simulink model "ctrl_TT"  (R2022b)
settings: Solver=FixedStepAuto  StartTime=0.0  StopTime=Tf  FixedStep=0.05  RelTol=1e-3
InitFcn:
  | run;
StopFcn:
  | save('testdata')
undefined symbols (not defined in the file): Ba_0, Bb, Bv_0, Bx_0, Cp, Cp_prime, d, dA_BP1, dA_BP2, dA_Hull, dA_PH, dA_Sail, dA_SProot, dA_X1a, dA_X1b, dA_X2a, dA_X2b, dA_X3a, dA_X3b, dA_X4a, dA_X4b, Ixx, Ixy, Ixz, Iyy, Iyz, Izz, Mb, n_BP1, n_BP2, n_Hull, n_PH, n_Sail, n_SProot, n_X2a, n_X2b, n_X3a, n_X4a, n_X4b, nt_BP1, nt_BP2, nt_Hull, nt_PH, nt_Sail, nt_SProot, nt_X1a, nt_X1b, nt_X2a, nt_X2b, nt_X3a, nt_X3b, nt_X4a, nt_X4b, Seastate, Tf, vt1_BP1, vt1_BP2, vt1_Hull, vt1_PH, vt1_Sail ... (+44)
libraries: simulink x8, sharedtransform x2, dspmathops x2
(part 1 of 5)
settings Model: Creator=yagkim  LastModifiedBy=maclin
settings SolverCC: AlgebraicLoopSolver=TrustRegion
settings DebuggingCC: UnconnectedInputMsg=warning  UnconnectedOutputMsg=warning  UnconnectedLineMsg=warning  SFMachineParentedDataDiag=warning  ArithmeticOperatorsInVariantConditions=warning
settings ModelReferenceCC: EnableRefExpFcnMdlSchedulingChecks=on
settings SFSimCC: CustomCodeUndefinedFunction=UseInterfaceOnly
settings RTWCC: DLArmComputeVersion=19.05

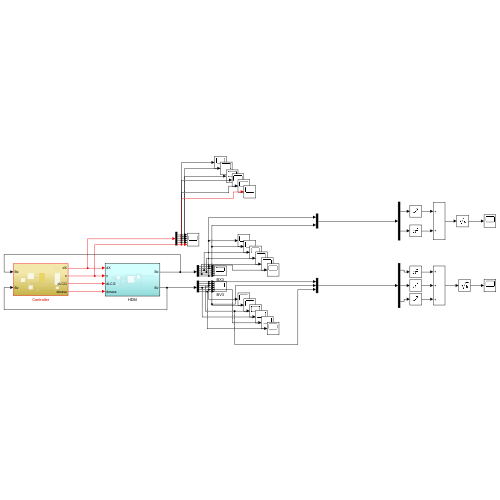
[thumbnail: Simulink's stored preview of the top-level diagram]
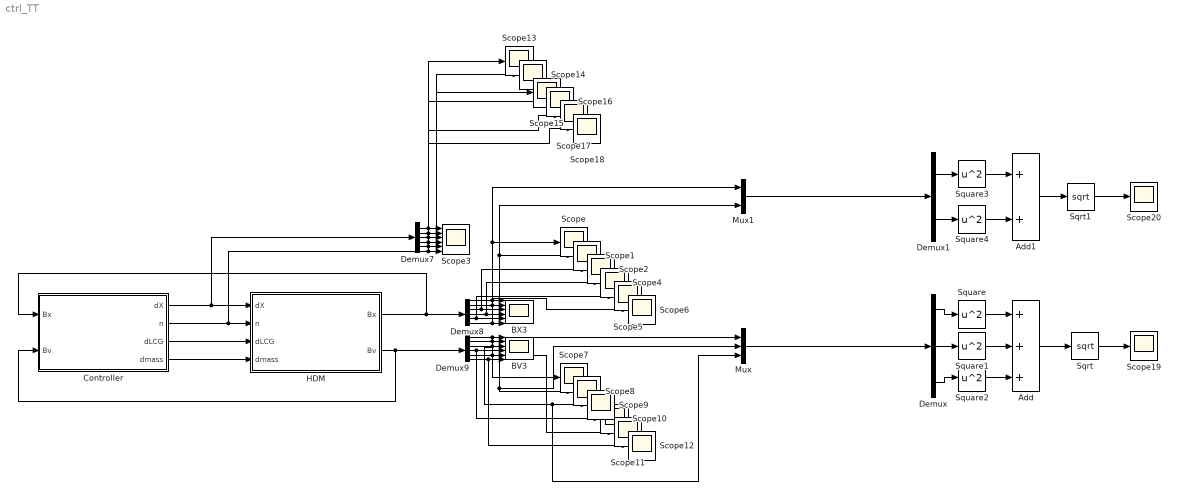
== system ctrl_TT ==
  Add : Sum  Inputs=+++
  Add1 : Sum
  BV3 : Scope  NumInputPorts=6
  BX3 : Scope  NumInputPorts=6
  Controller : Subsystem
  Demux : Demux  Outputs=3
  Demux1 : Demux  Outputs=2
  Demux7 : Demux  Outputs=5
  Demux8 : Demux  Outputs=6
  Demux9 : Demux  Outputs=6
  HDM : Subsystem
  Mux : Mux  Inputs=3
  Mux1 : Mux  Inputs=2
  Scope{,1..2,4..20} (20 alike) : Scope
  Scope3 : Scope  NumInputPorts=6
  Sqrt : Sqrt
  Sqrt1 : Sqrt
  Square{,1..4} (5 alike) : Math  Operator=square
  wires:
  Demux7/1 -> Scope13/1, Scope3/1
  Demux7/5 -> Scope17/1, Scope3/5
  Demux7/4 -> Scope16/1, Scope3/4
  Demux7/3 -> Scope15/1, Scope3/3
  Demux7/2 -> Scope14/1, Scope3/2
  Controller/4(dmass) -> HDM/4(dmass)
  Controller/3(dLCG) -> HDM/3(dLCG)
  Controller/1(dX) -> HDM/1(dX), Demux7/1
  Controller/2(n) -> HDM/2(n), Scope18/1, Scope3/6
  Demux8/1 -> Scope/1, Mux1/1, BX3/1
  Demux8/2 -> Scope1/1, Mux1/2, BX3/2
  Demux9/3 -> Mux/3, Scope9/1, BV3/3
  Demux8/3 -> BX3/3, Scope2/1
  Demux9/1 -> Mux/1, BV3/1, Scope7/1
  Demux8/4 -> BX3/4, Scope4/1
  Demux9/5 -> Scope11/1, BV3/5
  Demux8/6 -> Scope6/1, BX3/6
  Demux9/2 -> Mux/2, Scope8/1, BV3/2
  Demux8/5 -> BX3/5, Scope5/1
  Demux9/6 -> Scope12/1, BV3/6
  HDM/2(Bv) -> Controller/2(Bv), Demux9/1
  Demux9/4 -> BV3/4, Scope10/1
  HDM/1(Bx) -> Demux8/1, Controller/1(Bx)
  Add/1 -> Sqrt/1
  Square/1 -> Add/1
  Demux/1 -> Square/1
  Demux/3 -> Square2/1
  Sqrt/1 -> Scope19/1
  Square1/1 -> Add/2
  Square2/1 -> Add/3
  Demux/2 -> Square1/1
  Mux/1 -> Demux/1
  Square4/1 -> Add1/2
  Mux1/1 -> Demux1/1
  Sqrt1/1 -> Scope20/1
  Demux1/2 -> Square4/1
  Add1/1 -> Sqrt1/1
  Demux1/1 -> Square3/1
  Square3/1 -> Add1/1

== system ctrl_TT/Controller ==
  Bx : Inport
  Bv : Inport  Port=2
  Clock : Clock
  Constant : Constant  Value=[-1 0 0 0 0 0; 0 -1 0 0 0 0; 0 0 1 0 0 0; 0 0 0 1 0 0; 0 0 0 0 1 0; 0 0 0 0 0 1]
  Constant1 : Constant  Value=0
  Constant2 : Constant  Value=[-1 0 0 0 0 0; 0 -1 0 0 0 0; 0 0 1 0 0 0; 0 0 0 1 0 0; 0 0 0 0 1 0; 0 0 0 0 0 1]
  FF velocity ctrl : MATLAB Function  TreatAsAtomicUnit=on
  MATLAB Function2 : MATLAB Function  TreatAsAtomicUnit=on
  Marin PID : MATLAB Function  TreatAsAtomicUnit=on
  Matrix Multiply : Product  Multiplication=Matrix(*)
  Matrix Multiply1 : Product  Multiplication=Matrix(*)
  Scope : Scope
  Scope1 : Scope
  Selector1 : Selector  InputPortWidth=6  IndexOptions=Index vector (dialog)  Indices=[1 2 3]  OutputSizes=1
  Subsystem1 : Subsystem
  dX : Outport
  n : Outport  Port=2
  dLCG : Outport  Port=3
  dmass : Outport  Port=4
  wires:
  Subsystem1/1(z_d) -> Marin PID/1(z_ref)
  FF velocity ctrl/1(n) -> n/1
  Subsystem1/3(v) -> FF velocity ctrl/1(v_ref), Scope/1
  Marin PID/1(dX) -> dX/1
  Constant1/1 -> dLCG/1, dmass/1
  MATLAB Function2/1(pd) -> Scope1/1, Subsystem1/1(pd(t))
  MATLAB Function2/2(pdp) -> Subsystem1/2(pd(t)')
  Subsystem1/2(psi_d) -> Marin PID/2(psi_ref)
  Bx/1 -> Matrix Multiply/2
  Selector1/1 -> Subsystem1/3(p)
  Clock/1 -> MATLAB Function2/1(time)
  Matrix Multiply/1 -> Selector1/1, Marin PID/4(Bx)
  Constant/1 -> Matrix Multiply/1
  Bv/1 -> Matrix Multiply1/2
  Matrix Multiply1/1 -> Marin PID/3(Bv)
  Constant2/1 -> Matrix Multiply1/1

== system ctrl_TT/HDM ==
  dX : Inport
  n : Inport  Port=2
  dLCG : Inport  Port=3
  dmass : Inport  Port=4
  Constant1 : Constant  Value=Seastate
  HDM B3 : Subsystem  InitFcn='main'
  Integration and Coord. Transfrom : Subsystem
  Scope : Scope
  Scope1 : Scope
  actuator saturation : Subsystem
  Bx : Outport
  Bv : Outport  Port=2
  wires:
  actuator saturation/4(dmass (kg)) -> HDM B3/4(dmass), Scope1/1
  actuator saturation/3(dLCG (m)) -> HDM B3/3(dLCG)
  actuator saturation/2(n) -> HDM B3/2(n)
  actuator saturation/1(dX) -> HDM B3/1(dX CTRL)
  dmass/1 -> actuator saturation/4(dmass), Scope/1
  dLCG/1 -> actuator saturation/3(dLCG)
  n/1 -> actuator saturation/2("n ")
  dX/1 -> actuator saturation/1("dX ")
  Constant1/1 -> HDM B3/8(SeaState)
  HDM B3/1(F_hyd) -> Integration and Coord. Transfrom/2(F_hyd)
  Integration and Coord. Transfrom/3(Ba) -> HDM B3/7(Ba)
  Integration and Coord. Transfrom/1("Bx ") -> Bx/1, HDM B3/5(Bx), Integration and Coord. Transfrom/1(Bx)
  Integration and Coord. Transfrom/2(Bv) -> Bv/1, HDM B3/6(Bv)

== system ctrl_TT/Controller/Subsystem1 ==
  pd(t) : Inport
  pd(t)' : Inport  Port=2
  p : Inport  Port=3
  1,1 : Selector  NumberOfDimensions=2  InputPortWidth=3  IndexOptions=Index vector (dialog),Index vector (dialog)  Indices=1,1  OutputSizes=1,1
  2,1 : Selector  NumberOfDimensions=2  InputPortWidth=3  IndexOptions=Index vector (dialog),Index vector (dialog)  Indices=2,1  OutputSizes=1,1
  Add1 : Sum
  Demux3 : Demux  Outputs=3
  Derivative : Derivative
  Direction Cosine Matrix to Rotation Angles : sharedtransform/Direction Cosine Matrix to Rotation Angles  rotationOrder=ZYX  aMode=aMode  action=None  tolerance=eps(2)
      settings: LibrarySourceBlock=|
      | aerolibtransform2/Direction Cosine Matrix
      | to Rotation Angles
  Display{,1..7} (8 alike) : Display
  Dot Product1 : DotProduct  OutDataTypeStr=Inherit: Inherit via internal rule
  Gain : Gain  Gain=-1
  Gain1 : Gain  Gain=0.1
  MATLAB Function : MATLAB Function  TreatAsAtomicUnit=on
  Matrix Multiply1 : Product  Multiplication=Matrix(*)
  Mux1 : Mux  Inputs=2
  Scope : Scope
  Scope1 : Scope
  Selector : Selector  InputPortWidth=3  IndexOptions=Index vector (dialog)  Indices=[1 2]  OutputSizes=1
  Selector1 : Selector  InputPortWidth=3  IndexOptions=Index vector (dialog)  Indices=[1 2]  OutputSizes=1
  Subsystem1 : Subsystem
  Subsystem2 : Subsystem
  Subsystem3 : Subsystem
  Sum : Sum  Inputs=|+-
  Terminator3 : Terminator
  Terminator4 : Terminator
  z_d : Outport
  psi_d : Outport  Port=2
  v : Outport  Port=3
  wires:
  pd(t)'/1 -> Subsystem2/2(pd(y)'), Subsystem1/1(pd(t)'), Selector1/1
  pd(t)/1 -> Derivative/1, Sum/1, Subsystem2/1(pd(y))
  p/1 -> Sum/2, Subsystem2/3(p)
  Subsystem2/1(RTI) -> Matrix Multiply1/1, Display4/1
  2,1/1 -> Mux1/2
  1,1/1 -> Mux1/1
  Subsystem2/3(zd) -> z_d/1
  Gain/1 -> Display/1, psi_d/1
  Subsystem2/2(RWT) -> Matrix Multiply1/2
  Sum/1 -> Display6/1, Scope/1, Selector/1
  Derivative/1 -> Subsystem3/1(In1)
  Subsystem3/1(Out1) -> Scope1/1
  Gain1/1 -> Add1/1
  Add1/1 -> Dot Product1/1
  Mux1/1 -> Dot Product1/2
  Dot Product1/1 -> Display3/1, v/1
  Selector/1 -> Display5/1, Gain1/1
  Selector1/1 -> Add1/2
  Subsystem1/1(Out1) -> Display2/1
  Direction Cosine Matrix to Rotation Angles/1 -> Demux3/1
  Matrix Multiply1/1 -> MATLAB Function/1(u), Display7/1, 2,1/1, 1,1/1
  MATLAB Function/1(y) -> Display1/1, Direction Cosine Matrix to Rotation Angles/1
  Demux3/2 -> Terminator3/1
  Demux3/3 -> Terminator4/1
  Demux3/1 -> Gain/1

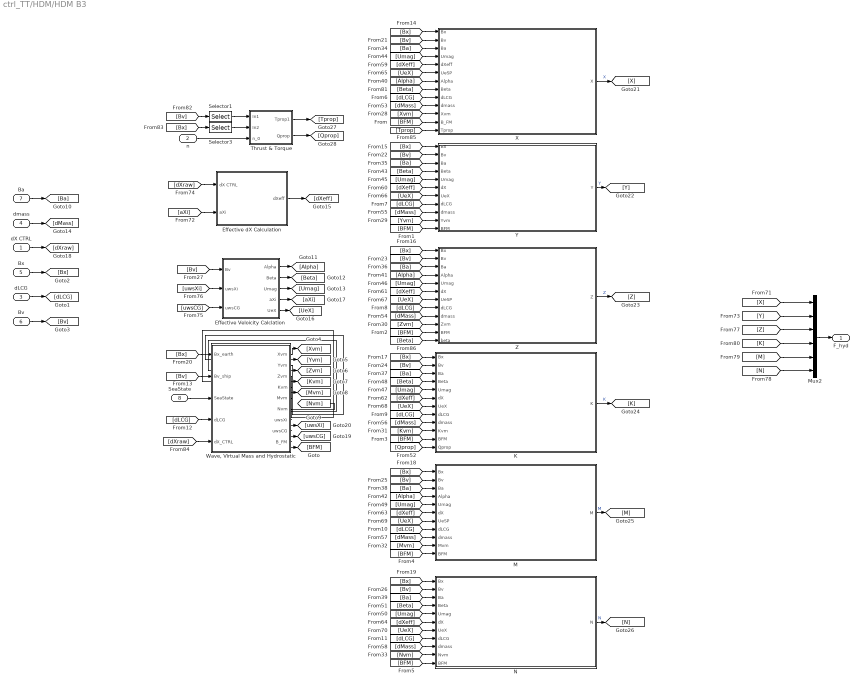
== system ctrl_TT/HDM/HDM B3 ==
  dX CTRL : Inport
  n : Inport  Port=2
  dLCG : Inport  Port=3
  dmass : Inport  Port=4
  Bx : Inport  Port=5
  Bv : Inport  Port=6
  Ba : Inport  Port=7
  SeaState : Inport  Port=8
  Effective Veloicity Calclation : Subsystem
  Effective dX Calculation : Subsystem
  K : Subsystem
  M : Subsystem
  Mux2 : Mux  Inputs=6
  N : Subsystem
  Selector1 : Selector  InputPortWidth=6  IndexOptions=Index vector (dialog)  Indices=1  OutputSizes=1
  Selector3 : Selector  InputPortWidth=6  IndexOptions=Index vector (dialog)  Indices=3  OutputSizes=1
  Thrust & Torque : Subsystem
  "Wave, Virtual Mass and Hydrostatic" : Subsystem
  X : Subsystem
  Y : Subsystem
  Z : Subsystem
  F_hyd : Outport  VectorParamsAs1DForOutWhenUnconnected=off
  wires:
  Z/1(Z) -> [Z]  "Z"
  [Beta] -> Z/12(beta)
  Thrust & Torque/2(Qprop) -> [Qprop]
  [Tprop] -> X/13(Tprop)
  Thrust & Torque/1(Tprop1) -> [Tprop]
  [Bx] -> Selector3/1
  Selector3/1 -> Thrust & Torque/2(In2)
  Selector1/1 -> Thrust & Torque/1(In1)
  [Bv] -> Selector1/1
  [Qprop] -> K/12(Qprop)
  [N] -> Mux2/6
  [M] -> Mux2/5
  [K] -> Mux2/4
  [Z] -> Mux2/3
  [Y] -> Mux2/2
  [X] -> Mux2/1
  [dXraw] -> "Wave, Virtual Mass and Hydrostatic"/5(dX_CTRL)
  [Beta] -> X/8(Beta)
  N/1(N) -> [N]  "N"
  M/1(M) -> [M]  "M"
  K/1(K) -> [K]  "K"
  Y/1(Y) -> [Y]  "Y"
  X/1(X) -> [X]  "X"
  [uwsXi] -> Effective Veloicity Calclation/2(uwsXi)
  "Wave, Virtual Mass and Hydrostatic"/7(uwsXi) -> [uwsXi]
  [uwsCG] -> Effective Veloicity Calclation/3(uwsCG)
  "Wave, Virtual Mass and Hydrostatic"/8(uwsCG) -> [uwsCG]
  [dXraw] -> Effective dX Calculation/1(dX CTRL)
  dX CTRL/1 -> [dXraw]
  [aXi] -> Effective dX Calculation/2(aXi)
  Effective Veloicity Calclation/4(aXi) -> [aXi]
  [UeX] -> N/7(UeX)
  [UeX] -> M/7(UeSP)
  [UeX] -> K/7(UeX)
  [UeX] -> Z/7(UeSP)
  [UeX] -> Y/7(UeX)
  [UeX] -> X/6(UeSP)
  Effective Veloicity Calclation/5(UeX) -> [UeX]
  [dXeff] -> N/6(dX)
  [dXeff] -> M/6(dX)
  [dXeff] -> K/6(dX)
  [dXeff] -> Z/6(dX)
  [dXeff] -> Y/6(dX)
  [dXeff] -> X/5(dXeff)
  [dMass] -> N/9(dmass)
  [dMass] -> M/9(dmass)
  [dMass] -> K/9(dmass)
  [dMass] -> Y/9(dmass)
  [dMass] -> Z/9(dmass)
  [dMass] -> X/10(dmass)
  dmass/1 -> [dMass]
  [Beta] -> N/4(Beta)
  [Umag] -> N/5(Umag)
  [Umag] -> M/5(Umag)
  [Beta] -> K/4(Beta)
  [Umag] -> K/5(Umag)
  [Umag] -> Z/5(Umag)
  [Umag] -> Y/5(Umag)
  [Umag] -> X/4(Umag)
  Effective Veloicity Calclation/3(Umag) -> [Umag]
  [Beta] -> Y/4(Beta)
  Effective Veloicity Calclation/2(Beta) -> [Beta]
  [Alpha] -> M/4(Alpha)
  [Alpha] -> Z/4(Alpha)
  [Alpha] -> X/7(Alpha)
  Effective Veloicity Calclation/1(Alpha) -> [Alpha]
  [Ba] -> N/3(Ba)
  [Ba] -> M/3(Ba)
  [Ba] -> K/3(Ba)
  [Ba] -> Z/3(Ba)
  [Ba] -> Y/3(Ba)
  [Ba] -> X/3(Ba)
  [Nvm] -> N/10(Nvm)
  [Mvm] -> M/10(Mvm)
  [Kvm] -> K/10(Kvm)
  [Bv] -> Z/2(Bv)
  [Zvm] -> Z/10(Zvm)
  [Yvm] -> Y/10(Yvm)
  [Xvm] -> X/11(Xvm)
  "Wave, Virtual Mass and Hydrostatic"/6(Nvm) -> [Nvm]
  "Wave, Virtual Mass and Hydrostatic"/5(Mvm) -> [Mvm]
  "Wave, Virtual Mass and Hydrostatic"/4(Kvm) -> [Kvm]
  "Wave, Virtual Mass and Hydrostatic"/3(Zvm) -> [Zvm]
  "Wave, Virtual Mass and Hydrostatic"/2(Yvm) -> [Yvm]
  "Wave, Virtual Mass and Hydrostatic"/1(Xvm) -> [Xvm]
  [Bv] -> Effective Veloicity Calclation/1(Bv)
  [Bv] -> N/2(Bv)
  [Bv] -> M/2(Bv)
  [Bv] -> K/2(Bv)
  [Bv] -> Y/2(Bv)
  [Bv] -> X/2(Bv)
  [Bv] -> "Wave, Virtual Mass and Hydrostatic"/2(Bv_ship)
  [Bx] -> "Wave, Virtual Mass and Hydrostatic"/1(Bx_earth)
  [Bx] -> N/1(Bx)
  [Bx] -> M/1(Bx)
  [Bx] -> K/1(Bx)
  [Bx] -> Z/1(Bx)
  [Bx] -> Y/1(Bx)
  [Bx] -> X/1(Bx)
  [dLCG] -> "Wave, Virtual Mass and Hydrostatic"/4(dLCG)
  [dLCG] -> N/8(dLCG)
  [dLCG] -> M/8(dLCG)
  [dLCG] -> K/8(dLCG)
  [dLCG] -> Z/8(dLCG)
  [dLCG] -> Y/8(dLCG)
  [dLCG] -> X/9(dLCG)
  [BFM] -> N/11(BFM)
  [BFM] -> M/11(BFM)
  [BFM] -> K/11(BFM)
  [BFM] -> Z/11(BFM)
  [BFM] -> Y/11(BFM)
  [BFM] -> X/12(B_FM)
  "Wave, Virtual Mass and Hydrostatic"/9(B_FM) -> [BFM]
  n/1 -> Thrust & Torque/3(n_0)
  SeaState/1 -> "Wave, Virtual Mass and Hydrostatic"/3(SeaState)
  Bv/1 -> [Bv]
  dLCG/1 -> [dLCG]
  Bx/1 -> [Bx]
  Ba/1 -> [Ba]
  Effective dX Calculation/1(dXeff) -> [dXeff]
  Mux2/1 -> F_hyd/1

== system ctrl_TT/HDM/Integration and Coord. Transfrom ==
  Bx : Inport
  F_hyd : Inport  Port=2
  Coordinate Transform : Subsystem
  Rigid Body Motion : Subsystem
  "Bx " : Outport
  Bv : Outport  Port=2
  Ba : Outport  Port=3
  wires:
  Bx/1 -> Rigid Body Motion/2(Bx)
  F_hyd/1 -> Rigid Body Motion/1(F_hyd)
  Rigid Body Motion/2(Ba) -> Ba/1
  Rigid Body Motion/1(Bv) -> Bv/1, Coordinate Transform/1(Bv)
  Coordinate Transform/1(X_earth) -> "Bx "/1

== system ctrl_TT/HDM/actuator saturation ==
  "dX " : Inport
  "n " : Inport  Port=2
  dLCG : Inport  Port=3
  dmass : Inport  Port=4
  " " : Subsystem
  "   " : Subsystem
  Subsystem1 : Subsystem
  Subsystem2 : Subsystem
  dX : Outport
  n : Outport  Port=2
  dLCG (m) : Outport  Port=3
  dmass (kg) : Outport  Port=4
  wires:
  "n "/1 -> "   "/1("n ")
  Subsystem2/1(dmass (kg)) -> dmass (kg)/1
  "dX "/1 -> " "/1("dX ")
  dmass/1 -> Subsystem2/1(dmass)
  Subsystem1/1(dLCG (m)) -> dLCG (m)/1
  dLCG/1 -> Subsystem1/1(dLCG)
  " "/1(dX) -> dX/1
  "   "/1(n) -> n/1

== system ctrl_TT/Controller/Subsystem1/Subsystem1 ==
  pd(t)' : Inport
  Add : Sum  Inputs=+++
  Demux : Demux  Outputs=3
  Sqrt : Sqrt
  Square : Math  Operator=square
  Square1 : Math  Operator=square
  Square2 : Math  Operator=square
  Out1 : Outport
  wires:
  Square2/1 -> Add/3
  Demux/3 -> Square2/1
  pd(t)'/1 -> Demux/1
  Demux/1 -> Square/1
  Demux/2 -> Square1/1
  Add/1 -> Sqrt/1
  Square/1 -> Add/1
  Square1/1 -> Add/2
  Sqrt/1 -> Out1/1

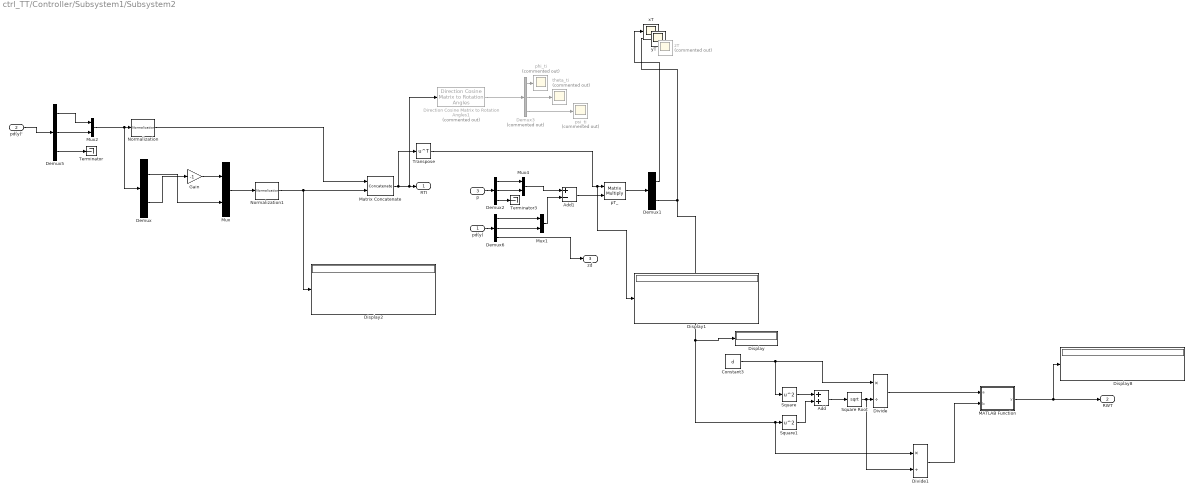
== system ctrl_TT/Controller/Subsystem1/Subsystem2 ==
  pd(y) : Inport
  pd(y)' : Inport  Port=2
  p : Inport  Port=3
  Add : Sum
  Add1 : Sum  Inputs=+-
  Constant3 : Constant  Value=d
  Demux : Demux  Outputs=2
  Demux1 : Demux  Outputs=2
  Demux2 : Demux  Outputs=3
  Demux3 : Demux  Commented=on  Outputs=3
  Demux5 : Demux  Outputs=3
  Demux6 : Demux  Outputs=3
  Direction Cosine Matrix to Rotation Angles1 : sharedtransform/Direction Cosine Matrix to Rotation Angles  Commented=on  rotationOrder=XYZ  aMode=aMode  action=None  tolerance=eps(2)
  Display{,1..2,8} (4 alike) : Display
  Divide : Product  Inputs=*/
  Divide1 : Product  Inputs=*/
  Gain : Gain  Gain=-1
  MATLAB Function : MATLAB Function  TreatAsAtomicUnit=on
  Matrix Concatenate : Concatenate  Mode=Multidimensional array  ConcatenateDimension=2
  Mux{,1..2,4} (4 alike) : Mux  Inputs=2
  Normalization : dspmathops/Normalization  NormType=2-norm  Bias=1e-10  NormOver=Each column  Dimension=1  roundingMode=Floor  overflowMode=off  accumDataTypeStr=Inherit: Same as product output  accumLastDataTypeStr=Inherit: Same as product output  outputDataTypeStr=Inherit: Same as product output  outputMin=[]  outputMax=[]  outputLastDataTypeStr=Inherit: Same as product output
  Normalization1 : dspmathops/Normalization  NormType=2-norm  Bias=1e-10  NormOver=Each column  Dimension=1  roundingMode=Floor  overflowMode=off  accumDataTypeStr=Inherit: Same as product output  accumLastDataTypeStr=Inherit: Same as product output  outputDataTypeStr=Inherit: Same as product output  outputMin=[]  outputMax=[]  outputLastDataTypeStr=Inherit: Same as product output
  Square : Math  Operator=square
  Square Root : Sqrt
  Square1 : Math  Operator=square
  Terminator : Terminator
  Terminator3 : Terminator
  Transpose : Math  Operator=transpose
  pT_ : Product  Multiplication=Matrix(*)
  phi_ti : Scope  Commented=on
  psi_ti : Scope  Commented=on
  theta_ti : Scope  Commented=on
  xT : Scope
  yT : Scope
  zT : Scope  Commented=on
  RTI : Outport
  RWT : Outport  Port=2
  zd : Outport  Port=3
  wires:
  Gain/1 -> Mux/1
  Demux/2 -> Gain/1
  Demux/1 -> Mux/2
  Mux/1 -> Normalization1/1
  Normalization/1 -> Matrix Concatenate/1
  Normalization1/1 -> Matrix Concatenate/2, Display2/1
  Matrix Concatenate/1 -> Direction Cosine Matrix to Rotation Angles1/1, RTI/1, Transpose/1
  Transpose/1 -> Display1/1, pT_/1
  Add1/1 -> pT_/2
  pT_/1 -> Demux1/1
  Demux1/2 -> yT/1, Display/1, Divide1/1, Square1/1
  Demux1/1 -> xT/1
  Direction Cosine Matrix to Rotation Angles1/1 -> Demux3/1
  Demux3/3 -> psi_ti/1
  Demux3/2 -> theta_ti/1
  Demux3/1 -> phi_ti/1
  Constant3/1 -> Square/1, Divide/1
  Square Root/1 -> Divide1/2, Divide/2
  Add/1 -> Square Root/1
  Square/1 -> Add/1
  Square1/1 -> Add/2
  Divide/1 -> MATLAB Function/1(a)
  Divide1/1 -> MATLAB Function/2(b)
  MATLAB Function/1(y) -> RWT/1, Display8/1
  Demux6/3 -> zd/1
  pd(y)'/1 -> Demux5/1
  Mux2/1 -> Demux/1, Normalization/1
  Demux5/1 -> Mux2/1
  Demux5/2 -> Mux2/2
  Demux5/3 -> Terminator/1
  Demux2/1 -> Mux4/1
  Demux2/3 -> Terminator3/1
  Demux2/2 -> Mux4/2
  Mux4/1 -> Add1/1
  p/1 -> Demux2/1
  Demux6/1 -> Mux1/1
  Demux6/2 -> Mux1/2
  pd(y)/1 -> Demux6/1
  Mux1/1 -> Add1/2

== system ctrl_TT/Controller/Subsystem1/Subsystem3 ==
  In1 : Inport
  Add : Sum  Inputs=+++
  Demux : Demux  Outputs=3
  Sqrt : Sqrt
  Square : Math  Operator=square
  Square1 : Math  Operator=square
  Square2 : Math  Operator=square
  Out1 : Outport
  wires:
  Sqrt/1 -> Out1/1
  Square1/1 -> Add/2
  Square/1 -> Add/1
  Add/1 -> Sqrt/1
  Demux/2 -> Square1/1
  Demux/1 -> Square/1
  In1/1 -> Demux/1
  Demux/3 -> Square2/1
  Square2/1 -> Add/3

== system ctrl_TT/HDM/HDM B3/Effective Veloicity Calclation ==
  Bv : Inport
  uwsXi : Inport  Port=2
  uwsCG : Inport  Port=3
  Add{,1..4} (5 alike) : Sum
  Demux : Demux  Outputs=5
  Demux1 : Demux  Outputs=3
  MATLAB Function : MATLAB Function  TreatAsAtomicUnit=on
  MATLAB Function1 : MATLAB Function  TreatAsAtomicUnit=on
  MATLAB Function2 : MATLAB Function  TreatAsAtomicUnit=on
  X_SP1 : Constant  Value=[31.924; 3.861; -3.861;]
  X_SP2 : Constant  Value=[31.924; 3.861; 3.861;]
  X_SP3 : Constant  Value=[31.924; -3.861; 3.861;]
  X_SP4 : Constant  Value=[31.924; -3.861; -3.861;]
  X_XB : Constant  Value=[-10.465; 0; 9.732;]
  n1 : Constant  Value=[0; 1/sqrt(2); -1/sqrt(2);]
  n2 : Constant  Value=[0; 1/sqrt(2); 1/sqrt(2);]
  n3 : Constant  Value=[0; -1/sqrt(2); 1/sqrt(2);]
  n4 : Constant  Value=[0; -1/sqrt(2); -1/sqrt(2);]
  n5 : Constant  Value=[0; 1; 0;]
  nh : Constant  Value=[-1; 0; 0;]
  Alpha : Outport
  Beta : Outport  Port=2
  Umag : Outport  Port=3
  aXi : Outport  Port=4
  UeX : Outport  Port=5
  wires:
  uwsXi/1 -> Demux/1
  MATLAB Function/1(aX) -> aXi/1
  MATLAB Function2/1(alpha) -> Alpha/1
  uwsCG/1 -> Demux1/1
  Demux1/3 -> MATLAB Function2/4(wCG)
  Demux1/2 -> MATLAB Function2/3(vCG)
  Demux1/1 -> MATLAB Function2/2(uCG)
  MATLAB Function/2(UeX) -> UeX/1
  MATLAB Function2/3(Umag) -> Umag/1
  MATLAB Function2/2(beta) -> Beta/1
  MATLAB Function1/2(urX2) -> Add1/1
  MATLAB Function1/3(urX3) -> Add2/1
  MATLAB Function1/4(urX4) -> Add3/1
  MATLAB Function1/5(urXB) -> Add4/1
  Demux/5 -> Add4/2
  Demux/4 -> Add3/2
  Demux/3 -> Add2/2
  Demux/2 -> Add1/2
  Add4/1 -> MATLAB Function/11(urXB)
  Add3/1 -> MATLAB Function/10(urX4)
  Add2/1 -> MATLAB Function/9(urX3)
  Add1/1 -> MATLAB Function/8(urX2)
  Add/1 -> MATLAB Function/7(urX1)
  Demux/1 -> Add/2
  MATLAB Function1/1(urX1) -> Add/1
  n5/1 -> MATLAB Function/6(nB)
  X_SP1/1 -> MATLAB Function1/1(rX1)
  X_SP4/1 -> MATLAB Function1/4(rX4)
  X_SP3/1 -> MATLAB Function1/3(rX3)
  X_SP2/1 -> MATLAB Function1/2(rX2)
  X_XB/1 -> MATLAB Function1/5(rXB)
  n4/1 -> MATLAB Function/5(n4)
  n3/1 -> MATLAB Function/4(n3)
  n2/1 -> MATLAB Function/3(n2)
  n1/1 -> MATLAB Function/2(n1)
  nh/1 -> MATLAB Function/1(nh)
  Bv/1 -> MATLAB Function2/1(Bv), MATLAB Function1/6(U_ship)

== system ctrl_TT/HDM/HDM B3/Effective dX Calculation ==
  dX CTRL : Inport
  aXi : Inport  Port=2
  Add{,1..4} (5 alike) : Sum
  Demux : Demux  Outputs=5
  Demux1 : Demux  Outputs=5
  Mux6 : Mux  Inputs=5
  dXeff : Outport
  wires:
  Mux6/1 -> dXeff/1
  Demux1/5 -> Add4/2
  Demux1/4 -> Add3/2
  Demux1/3 -> Add2/2
  Demux1/2 -> Add1/2
  Demux1/1 -> Add/2
  Demux/5 -> Add4/1
  Demux/4 -> Add3/1
  Demux/3 -> Add2/1
  Demux/2 -> Add1/1
  Demux/1 -> Add/1
  Add4/1 -> Mux6/5
  Add3/1 -> Mux6/4
  Add2/1 -> Mux6/3
  Add1/1 -> Mux6/2
  Add/1 -> Mux6/1
  aXi/1 -> Demux1/1
  dX CTRL/1 -> Demux/1

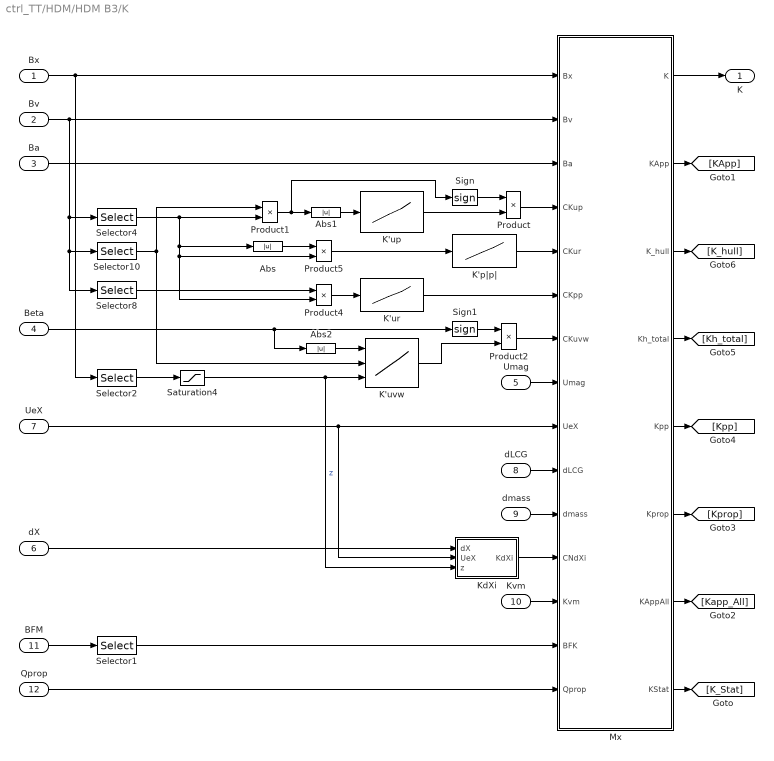
== system ctrl_TT/HDM/HDM B3/K ==
  Bx : Inport
  Bv : Inport  Port=2
  Ba : Inport  Port=3
  Beta : Inport  Port=4
  Umag : Inport  Port=5
  dX : Inport  Port=6
  UeX : Inport  Port=7
  dLCG : Inport  Port=8
  dmass : Inport  Port=9
  Kvm : Inport  Port=10
  BFM : Inport  Port=11
  Qprop : Inport  Port=12
  Abs : Abs  SaturateOnIntegerOverflow=off
  Abs1 : Abs  SaturateOnIntegerOverflow=off
  Abs2 : Abs  SaturateOnIntegerOverflow=off
  K'p|p| : Lookup_n-D  NumberOfTableDimensions=1  BreakpointsForDimension1=|  Table=|  InternalRulePriority=Speed  RndMeth=Simplest
      BreakpointsForDimension1=|
      | [-0.0015
      | -0.0012
      | -0.0009
      | -0.0006
      | -0.0003
      | -0.0001
      | 0.0001
      | 0.0003
      | 0.0006
      | 0.0009
      | 0.0012
      | 0.0015]
      Table=|
      | [-1.3011E-02
      | -1.6962E-02
      | -2.0682E-02
      | -3.1419E-02
      | -6.4407E-02
      | -1.9322E-01
      | 1.9322E-01
      | 6.4378E-02
      | 3.1944E-02
      | 2.1072E-02
      | 1.6415E-02
      | 1.3407E-02]
  K'up : Lookup_n-D  NumberOfTableDimensions=1  BreakpointsForDimension1=|  Table=|  InternalRulePriority=Speed  RndMeth=Simplest
      BreakpointsForDimension1=|
      | [0.03999989
      | 0.079999993
      | 0.11999963
      | 0.15999956]
      Table=|
      | [-4.0344E-04
      | -8.1402E-04
      | -1.2116E-03
      | -1.6125E-03]
  K'ur : Lookup_n-D  NumberOfTableDimensions=1  BreakpointsForDimension1=|  Table=|  InternalRulePriority=Speed  RndMeth=Simplest
      BreakpointsForDimension1=|
      | [-0.0015
      | -0.0012
      | -0.0009
      | -0.0006
      | -0.0003
      | -0.0001
      | 0.0001
      | 0.0003
      | 0.0006
      | 0.0009
      | 0.0012
      | 0.0015]
      Table=|
      | [-1.3011E-02
      | -1.6962E-02
      | -2.0682E-02
      | -3.1419E-02
      | -6.4407E-02
      | -1.9322E-01
      | 1.9322E-01
      | 6.4378E-02
      | 3.1944E-02
      | 2.1072E-02
      | 1.6415E-02
      | 1.3407E-02]
  K'uvw : Lookup_n-D  NumberOfTableDimensions=3  BreakpointsForDimension1=|  BreakpointsForDimension2=|  BreakpointsForDimension3=|  Table=|  InternalRulePriority=Speed  RndMeth=Simplest
      BreakpointsForDimension1=|
      | [0
      | 4
      | 8
      | 12]
      BreakpointsForDimension2=|
      | [-5.1444E+00
      | -3.0866E+00
      | -1.5433E+00
      | ]
      Table=|
      | reshape([0.0000000E+00
      | 1.5570290E-04
      | 3.7677829E-04
      | 6.0025374E-04
      | 0.0000000E+00
      | 1.5575678E-04
      | 3.8557685E-04
      | 6.0103850E-04
      | 0.0000000E+00
      | 1.7511088E-04
      | 3.8376789E-04
      | 6.0108480E-04
      | 0.0000000E+00
      | 1.9071552E-04
      | 4.0986649E-04
      | 6.4012030E-04
      | 0.0000000E+00
      | 1.8940622E-04
      | 4.0946931E-04
      | 6.3613461E-04
      | 0.0000000E+00
      | 1.8621071E-04
      | 4.0619654E-04
      | 7.0286379E-04
      | 0.0000000E+00
      | 2.0712189E-04
      | 4.4751988E-04
      | 7.0514631E-04
      | 0.0000000E+00
      | 1.9895751E-04
      | 4.3099356E-04
      | 6.6994571E-04
      | 0.0000000E+00
      | 1.9568554E-04
      | 4.2679977E-04
      | 6.6445067E-04
      | 0.0000000E+00
      | 2.4359563E-04
      | 5.3740096E-04
      | 8.5879902E-04
      | 0.0000000E+00
      | 2.0890025E-04
      | 4.5502130E-04
      | 7.1388224E-04
      | 0.0000000E+00
      | 2.0575072E-04
      | 4.5505766E-04
      | 7.0285206E-04],[4,3,4])
      BreakpointsForDimension3=|
      | [-35.0624 -18.3724 -15.3724 -13.8724
      | ]
      settings: InputPortMap=u0,u1,u2
  KdXi : Subsystem
  Mx : MATLAB Function  TreatAsAtomicUnit=on
  Product{,1..2,4..5} (5 alike) : Product
  Saturation4 : Saturate  UpperLimit=-13.8724  LowerLimit=-35.0624
  Selector1 : Selector  InputPortWidth=6  IndexOptions=Index vector (dialog)  Indices=4  OutputSizes=1
  Selector10 : Selector  InputPortWidth=6  IndexOptions=Index vector (dialog)  Indices=1  OutputSizes=1
  Selector2 : Selector  InputPortWidth=6  IndexOptions=Index vector (dialog)  Indices=3  OutputSizes=1
  Selector4 : Selector  InputPortWidth=6  IndexOptions=Index vector (dialog)  Indices=4  OutputSizes=1
  Selector8 : Selector  InputPortWidth=6  IndexOptions=Index vector (dialog)  Indices=2  OutputSizes=1
  Sign : Signum
  Sign1 : Signum
  K : Outport
  wires:
  Mx/3(K_hull) -> [K_hull]
  Mx/4(Kh_total) -> [Kh_total]
  Mx/5(Kpp) -> [Kpp]
  Mx/6(Kprop) -> [Kprop]
  Mx/7(KAppAll) -> [Kapp_All]
  Mx/2(KApp) -> [KApp]
  Qprop/1 -> Mx/15(Qprop)
  Kvm/1 -> Mx/13(Kvm)
  Saturation4/1 -> K'uvw/3, KdXi/3(z)  "z"
  K'p|p|/1 -> Mx/5(CKur)
  Product/1 -> Mx/4(CKup)
  Sign1/1 -> Product2/1
  Mx/8(KStat) -> [K_Stat]
  Mx/1(K) -> K/1
  Selector1/1 -> Mx/14(BFK)
  BFM/1 -> Selector1/1
  Abs2/1 -> K'uvw/1
  Product2/1 -> Mx/7(CKuvw)
  Sign/1 -> Product/1
  Abs1/1 -> K'up/1
  Product1/1 -> Abs1/1, Sign/1
  K'uvw/1 -> Product2/2
  Selector2/1 -> Saturation4/1
  KdXi/1(KdXi) -> Mx/12(CNdXi)
  K'ur/1 -> Mx/6(CKpp)
  Selector4/1 -> Product1/2, Abs/1, Product5/2, Product4/2
  Product5/1 -> K'p|p|/1
  Abs/1 -> Product5/1
  Selector8/1 -> Product4/1
  Product4/1 -> K'ur/1
  K'up/1 -> Product/2
  dX/1 -> KdXi/1(dX)
  dmass/1 -> Mx/11(dmass)
  dLCG/1 -> Mx/10(dLCG)
  Umag/1 -> Mx/8(Umag)
  Beta/1 -> Sign1/1, Abs2/1
  UeX/1 -> KdXi/2(UeX), Mx/9(UeX)
  Ba/1 -> Mx/3(Ba)
  Selector10/1 -> Product1/1, K'uvw/2
  Bx/1 -> Selector2/1, Mx/1(Bx)
  Bv/1 -> Mx/2(Bv), Selector4/1, Selector10/1, Selector8/1

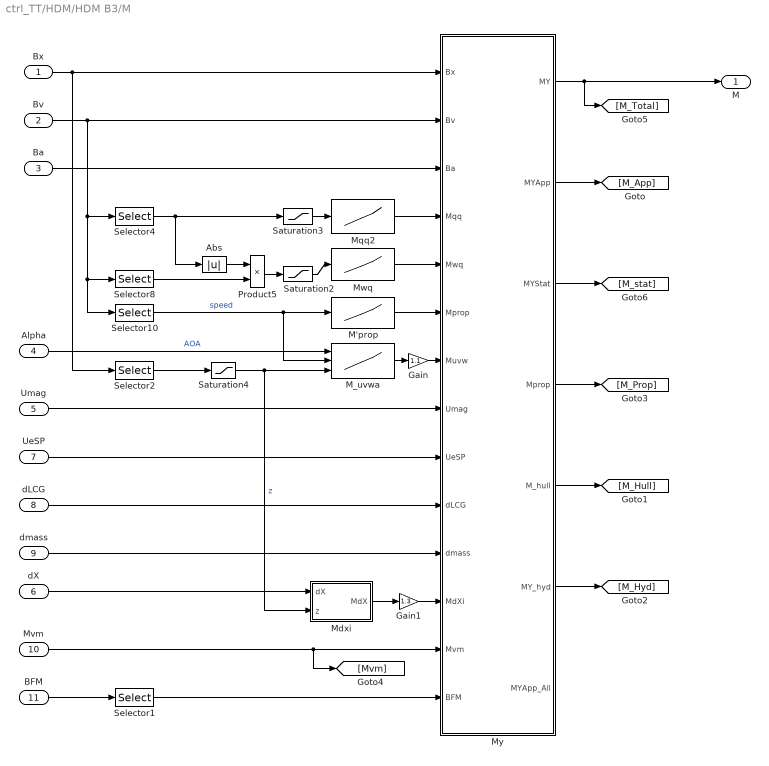
== system ctrl_TT/HDM/HDM B3/M ==
  Bx : Inport
  Bv : Inport  Port=2
  Ba : Inport  Port=3
  Alpha : Inport  Port=4
  Umag : Inport  Port=5
  dX : Inport  Port=6
  UeSP : Inport  Port=7
  dLCG : Inport  Port=8
  dmass : Inport  Port=9
  Mvm : Inport  Port=10
  BFM : Inport  Port=11
  Abs : Abs  SaturateOnIntegerOverflow=off
  Gain : Gain  Gain=1.1
  Gain1 : Gain  Gain=1.3
  M'prop : Lookup_n-D  NumberOfTableDimensions=1  BreakpointsForDimension1=[-7.7166666 -5.1444444 -3.08666664]  Table=[-0.00022 -0.0002 -0.00015]  InternalRulePriority=Speed  RndMeth=Simplest
  M_uvwa : Lookup_n-D  NumberOfTableDimensions=3  BreakpointsForDimension1=|  BreakpointsForDimension2=|  BreakpointsForDimension3=|  Table=|  InternalRulePriority=Speed  RndMeth=Simplest
      BreakpointsForDimension1=|
      | [-12
      | -8
      | -4
      | 0
      | 4
      | 8
      | 12]
      BreakpointsForDimension2=|
      | [-5.1444E+00
      | -3.0866E+00
      | -1.5433E+00
      | ]
      Table=|
      | reshape([-2.40251E-03
      | -1.59538E-03
      | -8.21748E-04
      | -3.60182E-06
      | 8.13350E-04
      | 1.50586E-03
      | 2.39707E-03
      | -2.43392E-03
      | -1.61509E-03
      | -8.50748E-04
      | -3.60182E-06
      | 8.24271E-04
      | 1.51842E-03
      | 2.43805E-03
      | -2.45014E-03
      | -1.65711E-03
      | -9.11210E-04
      | -3.60182E-06
      | 8.61300E-04
      | 1.57459E-03
      | 2.42777E-03
      | -2.54380E-03
      | -1.68842E-03
      | -8.33041E-04
      | 2.23377E-05
      | 8.77717E-04
      | 1.73310E-03
      | 2.58847E-03
      | -2.63734E-03
      | -1.75078E-03
      | -8.64221E-04
      | 2.23377E-05
      | 9.08896E-04
      | 1.79546E-03
      | 2.68201E-03
      | -2.83738E-03
      | -1.88414E-03
      | -9.30902E-04
      | 2.23377E-05
      | 9.75577E-04
      | 1.92882E-03
      | 2.88206E-03
      | -2.63786E-03
      | -1.74504E-03
      | -8.52211E-04
      | 4.06140E-05
      | 9.33439E-04
      | 1.82626E-03
      | 2.71909E-03
      | -2.63728E-03
      | -1.74465E-03
      | -8.52017E-04
      | 4.06140E-05
      | 9.33245E-04
      | 1.82588E-03
      | 2.71851E-03
      | -2.86138E-03
      | -1.89405E-03
      | -9.26716E-04
      | 4.06140E-05
      | 1.00794E-03
      | 1.97527E-03
      | 2.94260E-03
      | -0.002723494
      | -0.001792522
      | -0.000861549
      | 6.9423E-05
      | 0.001000396
      | 0.001931368
      | 0.002862341
      | -0.002736476
      | -0.001798489
      | -0.000860502
      | 6.9423E-05
      | 0.001015473
      | 0.00195346
      | 0.002891447
      | -0.002765582
      | -0.00182058
      | -0.000875579
      | 6.9423E-05
      | 0.001014425
      | 0.001959426
      | 0.002904428],[7,3,4])
      BreakpointsForDimension3=|
      | [-35.0624 -18.3724 -15.3724 -13.8724
      | ]
      settings: InputPortMap=u0,u1,u2
  Mdxi : Subsystem
  Mqq2 : Lookup_n-D  NumberOfTableDimensions=1  BreakpointsForDimension1=|  Table=|  InternalRulePriority=Speed  RndMeth=Simplest
      BreakpointsForDimension1=|
      | [-0.02
      | -0.015
      | -0.012958963
      | -0.009719222
      | -0.006479482
      | -0.003239741
      | -0.00161987
      | -0.000647948
      | 0.000647948
      | 0.00161987
      | 0.003239741
      | 0.006479482
      | 0.009719222
      | 0.012958963
      | 0.015
      | 0.02
      | ]
      Table=|
      | [-2.2571E-03
      | -2.3029E-03
      | -2.0965E-03
      | -2.0229E-03
      | -2.1546E-03
      | -1.4789E-03
      | -1.5664E-03
      | -1.4544E-03
      | -1.4705E-03
      | -1.4942E-03
      | -1.8790E-03
      | -1.8821E-03
      | -2.1009E-03
      | -2.0521E-03
      | -2.1685E-03
      | -2.0822E-03
      | ]
  Mwq : Lookup_n-D  NumberOfTableDimensions=1  BreakpointsForDimension1=|  Table=|  InternalRulePriority=Speed  RndMeth=Simplest
      BreakpointsForDimension1=|
      | [-0.0015
      | -0.0012
      | -0.0009
      | -0.0006
      | -0.0003
      | -0.0001
      | 0.0001
      | 0.0003
      | 0.0006
      | 0.0009
      | 0.0012
      | 0.0015]
      Table=|
      | [-1.3011E-02
      | -1.6962E-02
      | -2.0682E-02
      | -3.1419E-02
      | -6.4407E-02
      | -1.9322E-01
      | 1.9322E-01
      | 6.4378E-02
      | 3.1944E-02
      | 2.1072E-02
      | 1.6415E-02
      | 1.3407E-02]
  My : MATLAB Function  TreatAsAtomicUnit=on
  Product5 : Product
  Saturation2 : Saturate  UpperLimit=0.0015  LowerLimit=-0.0015
  Saturation3 : Saturate  UpperLimit=0.02  LowerLimit=-0.02
  Saturation4 : Saturate  UpperLimit=-13.8724  LowerLimit=-35.0624
  Selector1 : Selector  InputPortWidth=6  IndexOptions=Index vector (dialog)  Indices=5  OutputSizes=1
  Selector10 : Selector  InputPortWidth=6  IndexOptions=Index vector (dialog)  Indices=1  OutputSizes=1
  Selector2 : Selector  InputPortWidth=6  IndexOptions=Index vector (dialog)  Indices=3  OutputSizes=1
  Selector4 : Selector  InputPortWidth=6  IndexOptions=Index vector (dialog)  Indices=5  OutputSizes=1
  Selector8 : Selector  InputPortWidth=6  IndexOptions=Index vector (dialog)  Indices=3  OutputSizes=1
  M : Outport
  wires:
  Gain1/1 -> My/12(MdXi)
  My/4(Mprop) -> [M_Prop]
  My/6(MY_hyd) -> [M_Hyd]
  My/5(M_hull) -> [M_Hull]
  My/2(MYApp) -> [M_App]
  Selector1/1 -> My/14(BFM)
  BFM/1 -> Selector1/1
  Gain/1 -> My/7(Muvw)
  Saturation4/1 -> M_uvwa/3, Mdxi/2(z)  "z"
  My/3(MYStat) -> [M_stat]
  Bv/1 -> My/2(Bv), Selector4/1, Selector8/1, Selector10/1
  Bx/1 -> My/1(Bx), Selector2/1
  Selector10/1 -> M'prop/1, M_uvwa/2  "speed"
  Ba/1 -> My/3(Ba)
  M'prop/1 -> My/6("Mprop ")
  UeSP/1 -> My/9(UeSP)
  Selector4/1 -> Saturation3/1, Abs/1
  Alpha/1 -> M_uvwa/1  "AOA"
  Umag/1 -> My/8(Umag)
  dLCG/1 -> My/10(dLCG)
  dmass/1 -> My/11(dmass)
  dX/1 -> Mdxi/1(dX)
  Mqq2/1 -> My/4(Mqq)
  Mwq/1 -> My/5(Mwq)
  Product5/1 -> Saturation2/1
  Selector8/1 -> Product5/2
  Abs/1 -> Product5/1
  Saturation2/1 -> Mwq/1
  Saturation3/1 -> Mqq2/1
  My/1(MY) -> [M_Total], M/1
  Mdxi/1(MdX) -> Gain1/1
  Mvm/1 -> [Mvm], My/13(Mvm)
  Selector2/1 -> Saturation4/1
  M_uvwa/1 -> Gain/1

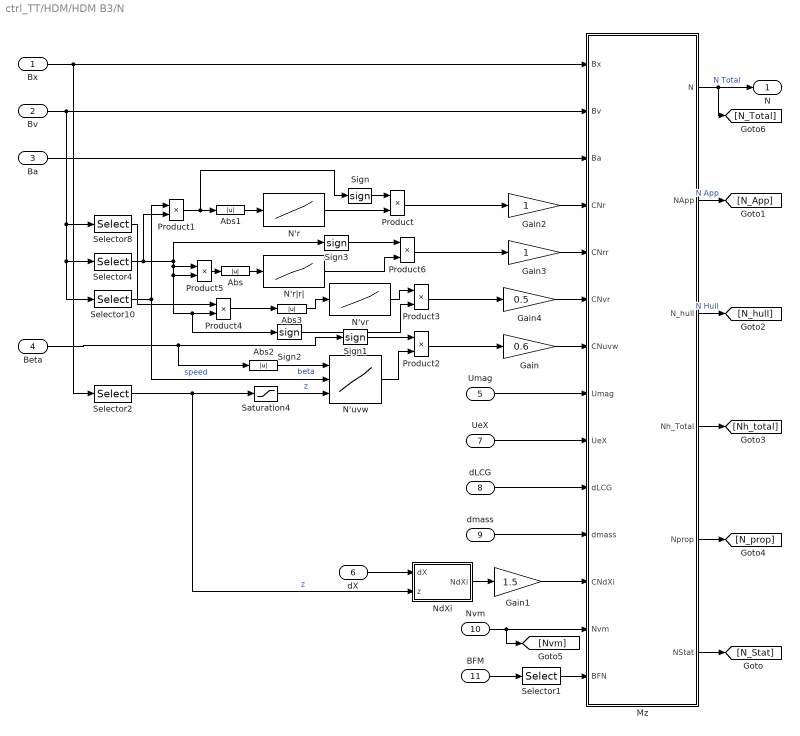
== system ctrl_TT/HDM/HDM B3/N ==
  Bx : Inport
  Bv : Inport  Port=2
  Ba : Inport  Port=3
  Beta : Inport  Port=4
  Umag : Inport  Port=5
  dX : Inport  Port=6
  UeX : Inport  Port=7
  dLCG : Inport  Port=8
  dmass : Inport  Port=9
  Nvm : Inport  Port=10
  BFM : Inport  Port=11
  Abs{,1..3} (4 alike) : Abs  SaturateOnIntegerOverflow=off
  Gain : Gain  Gain=0.6
  Gain1 : Gain  Gain=1.5
  Gain2 : Gain
  Gain3 : Gain
  Gain4 : Gain  Gain=0.5
  Mz : MATLAB Function  TreatAsAtomicUnit=on
  N'r : Lookup_n-D  NumberOfTableDimensions=1  BreakpointsForDimension1=|  Table=|  InternalRulePriority=Speed  RndMeth=Simplest
      BreakpointsForDimension1=|
      | [0.03999989
      | 0.079999993
      | 0.11999963
      | 0.15999956]
      Table=|
      | [-4.0344E-04
      | -8.1402E-04
      | -1.2116E-03
      | -1.6125E-03]
  N'r|r| : Lookup_n-D  NumberOfTableDimensions=1  BreakpointsForDimension1=|  Table=|  InternalRulePriority=Speed  RndMeth=Simplest
      BreakpointsForDimension1=|
      | [0.0001
      | 0.0003
      | 0.0006
      | 0.0009
      | 0.0012
      | 0.0015
      | ]
      Table=|
      | [1.93E-01
      | 6.44E-02
      | 3.19E-02
      | 2.11E-02
      | 1.64E-02
      | 1.34E-02
      | ]
  N'uvw : Lookup_n-D  NumberOfTableDimensions=3  BreakpointsForDimension1=|  BreakpointsForDimension2=|  BreakpointsForDimension3=|  Table=|  InternalRulePriority=Speed  RndMeth=Simplest
      BreakpointsForDimension1=|
      | [0
      | 4
      | 8
      | 12]
      BreakpointsForDimension2=|
      | [-5.1444E+00
      | -3.0866E+00
      | -1.5433E+00
      | ]
      Table=|
      | reshape([0.0000000E+00
      | 1.1975814E-03
      | 2.7970643E-03
      | 4.1308534E-03
      | 0.0000000E+00
      | 1.2111628E-03
      | 2.9207146E-03
      | 4.1207837E-03
      | 0.0000000E+00
      | 1.4959851E-03
      | 2.9486406E-03
      | 4.1213058E-03
      | 0.0000000E+00
      | 1.4879743E-03
      | 2.9975710E-03
      | 4.2577903E-03
      | 0.0000000E+00
      | 1.4933232E-03
      | 3.0017417E-03
      | 4.2334501E-03
      | 0.0000000E+00
      | 1.5365285E-03
      | 3.0446384E-03
      | 4.4091424E-03
      | 0.0000000E+00
      | 1.5329300E-03
      | 3.0664177E-03
      | 4.3937198E-03
      | 0.0000000E+00
      | 1.5274021E-03
      | 3.0742094E-03
      | 4.3066710E-03
      | 0.0000000E+00
      | 1.5692494E-03
      | 3.1052278E-03
      | 4.3211963E-03
      | 0.0000000E+00
      | 1.5996020E-03
      | 3.2227652E-03
      | 4.5425478E-03
      | 0.0000000E+00
      | 1.5650123E-03
      | 3.1236229E-03
      | 4.4022471E-03
      | 0.0000000E+00
      | 1.6041810E-03
      | 3.1241151E-03
      | 4.4103656E-03],[4,3,4])
      BreakpointsForDimension3=|
      | [-35.0624 -18.3724 -15.3724 -13.8724
      | ]
      settings: InputPortMap=u0,u1,u2
  N'vr : Lookup_n-D  NumberOfTableDimensions=1  BreakpointsForDimension1=|  Table=|  InternalRulePriority=Speed  RndMeth=Simplest
      BreakpointsForDimension1=|
      | [0
      | 0.051444
      | 0.102888
      | 0.205776
      | 0.411552]
      Table=|
      | [0.0000E+00
      | -1.9921E-03
      | -9.2025E-03
      | -3.2154E-02
      | -1.3255E-01]
  NdXi : Subsystem
  Product{,1..6} (7 alike) : Product
  Saturation4 : Saturate  UpperLimit=-13.8724  LowerLimit=-35.0624
  Selector1 : Selector  InputPortWidth=6  IndexOptions=Index vector (dialog)  Indices=6  OutputSizes=1
  Selector10 : Selector  InputPortWidth=6  IndexOptions=Index vector (dialog)  Indices=1  OutputSizes=1
  Selector2 : Selector  InputPortWidth=6  IndexOptions=Index vector (dialog)  Indices=3  OutputSizes=1
  Selector4 : Selector  InputPortWidth=6  IndexOptions=Index vector (dialog)  Indices=6  OutputSizes=1
  Selector8 : Selector  InputPortWidth=6  IndexOptions=Index vector (dialog)  Indices=2  OutputSizes=1
  Sign{,1..3} (4 alike) : Signum
  N : Outport
  wires:
  Mz/5(Nprop) -> [N_prop]
  Mz/4(Nh_Total) -> [Nh_total]
  Mz/3(N_hull) -> [N_hull]  "N Hull"
  Mz/2(NApp) -> [N_App]  "N App"
  Abs/1 -> N'r|r|/1
  Sign3/1 -> Product6/1
  Product6/1 -> Gain3/1
  Sign2/1 -> Product3/2
  N'vr/1 -> Product3/1
  Abs3/1 -> N'vr/1
  Saturation4/1 -> N'uvw/3  "z"
  Gain4/1 -> Mz/6(CNvr)
  Gain3/1 -> Mz/5(CNrr)
  Gain2/1 -> Mz/4(CNr)
  Mz/6(NStat) -> [N_Stat]
  Selector1/1 -> Mz/14(BFN)
  BFM/1 -> Selector1/1
  Nvm/1 -> [Nvm], Mz/13(Nvm)
  Gain1/1 -> Mz/12(CNdXi)
  NdXi/1(NdXi) -> Gain1/1
  Gain/1 -> Mz/7(CNuvw)
  Product2/1 -> Gain/1
  Sign1/1 -> Product2/1
  Abs2/1 -> N'uvw/1  "beta"
  Product/1 -> Gain2/1
  Sign/1 -> Product/1
  Abs1/1 -> N'r/1
  Product1/1 -> Abs1/1, Sign/1
  N'uvw/1 -> Product2/2
  Selector2/1 -> Saturation4/1, NdXi/2(z)  "z"
  Mz/1(N) -> [N_Total], N/1  "N Total"
  Product3/1 -> Gain4/1
  Product5/1 -> Abs/1
  Selector4/1 -> Product1/2, Sign3/1, Product5/2, Sign2/1, Product4/2, Product5/1
  Selector8/1 -> Product4/1
  Product4/1 -> Abs3/1
  N'r|r|/1 -> Product6/2
  N'r/1 -> Product/2
  dX/1 -> NdXi/1(dX)
  dmass/1 -> Mz/11(dmass)
  dLCG/1 -> Mz/10(dLCG)
  Umag/1 -> Mz/8(Umag)
  Beta/1 -> Sign1/1, Abs2/1
  UeX/1 -> Mz/9(UeX)
  Ba/1 -> Mz/3(Ba)
  Selector10/1 -> Product1/1, N'uvw/2  "speed"
  Bx/1 -> Mz/1(Bx), Selector2/1
  Bv/1 -> Mz/2(Bv), Selector8/1, Selector4/1, Selector10/1

== system ctrl_TT/HDM/HDM B3/Thrust & Torque ==
  In1 : Inport
  In2 : Inport  Port=2
  n_0 : Inport  Port=3
  Gain20 : Gain  Gain=-1
  Saturation5 : Saturate  UpperLimit=-13.8724  LowerLimit=-36.3724
  Saturation7 : Saturate  UpperLimit=-1.54333333  LowerLimit=-5.14444
  "Thrust Deduction, 25m1" : Lookup_n-D  BreakpointsForDimension1=|  BreakpointsForDimension2=[-5.14444 -3.086664 -1.543332]  Table=|  InternalRulePriority=Speed  RndMeth=Simplest
      BreakpointsForDimension1=|
      | [-36.3724
      | -18.3724
      | -15.3724
      | -13.8724]
      Table=|
      | reshape([0.245958
      | 0.251311246
      | 0.25251
      | 0.251322
      | 0.2444134
      | 0.2498597
      | 0.2509219
      | 0.2498992
      | 0.2496
      | 0.2594532
      | 0.257802
      | 0.2475762],[4,3])
      settings: InputPortMap=u0,u1
  Tprop : MATLAB Function  TreatAsAtomicUnit=on
  Tprop1 : Outport
  Qprop : Outport  Port=2
  wires:
  n_0/1 -> Tprop/3(n_0)
  Saturation7/1 -> "Thrust Deduction, 25m1"/2
  Tprop/2(Qprop) -> Qprop/1
  Gain20/1 -> Tprop/1(speed)
  Saturation5/1 -> "Thrust Deduction, 25m1"/1
  "Thrust Deduction, 25m1"/1 -> Tprop/2(Td)
  Tprop/1(Tprop) -> Tprop1/1
  In2/1 -> Saturation7/1
  In1/1 -> Gain20/1, Saturation5/1

== system ctrl_TT/HDM/HDM B3/Wave, Virtual Mass and Hydrostatic ==
  Bx_earth : Inport
  Bv_ship : Inport  Port=2
  SeaState : Inport  Port=3
  dLCG : Inport  Port=4
  dX_CTRL : Inport  Port=5
  Add : Sum  Inputs=+-
  CG : Constant  Value=Xcg
  CGi : Constant  Value=|
      | [5.0784E+00	0.0000E+00	8.0728E-03;
      | 1.1013E+01	0.0000E+00	2.5384E-01;
      | 1.7302E+01	0.0000E+00	3.0728E-01;
      | 2.5741E+01	0.0000E+00	4.1417E-01;
      | 3.4688E+01	0.0000E+00	4.1585E-01;
      | 4.2324E+01	0.0000E+00	3.2444E-01;
      | 4.9992E+01	0.0000E+00	3.3454E-01;
      | 5.7427E+01	0.0000E+00	1.7420E-02;
      | 6.3078E+01	0.0000E+00	1.8824E-02;
      | 6.6703E+01	0.0000E+00	1.1340E-02;
      | 2.5141E+01	0.0000E+00	8.6491E+00;
      | 2.1732E+01	0.0000E+00	9.7273E+00;
      | 6.3166E+01	0.0000E+00	-4.0823E-17;
      | 2.2043E+01	0.0000E+00	9.7261E+00;
      | 6.3451E+01	0.0000E+00	-6.2238E-17;
      | ]
  Cvm*dm : Constant  Value=|
      | [8.4658E+04	1.7229E+05	1.6487E+05
      | 2.3551E+04	4.3394E+05	3.6176E+05
      | 1.1585E+03	5.9767E+05	4.2996E+05
      | 1.4123E+02	1.1354E+06	6.5606E+05
      | 9.1503E+01	6.9712E+05	5.1688E+05
      | 9.6110E+01	6.7201E+05	5.1905E+05
      | 1.2163E+04	5.7818E+05	4.7547E+05
      | 3.7219E+04	3.4697E+05	3.3508E+05
      | 1.9318E+04	7.7284E+04	7.6560E+04
      | 1.5368E+04	2.6375E+04	2.6268E+04
      | 1.8312E+04	4.5870E+05	5.1108E+04
      | 3.1859E+02	1.2645E+04	3.4886E+02
      | 3.0285E+03	4.4945E+04	4.4489E+04
      | 7.9160E+02	8.8963E+02	1.3306E+04
      | 1.2115E+03	3.9547E+04	3.9205E+04
      | ]
  Demux : Demux  Outputs=3
  Demux1 : Demux  Outputs=3
  Derivative1 : Derivative
  MATLAB Function : MATLAB Function  TreatAsAtomicUnit=on
  Wave Particle Motions : Subsystem
  beta_wave : Constant  Value=0
  phi_wave : Constant  Value=0
  Xvm : Outport
  Yvm : Outport  Port=2
  Zvm : Outport  Port=3
  Kvm : Outport  Port=4
  Mvm : Outport  Port=5
  Nvm : Outport  Port=6
  uwsXi : Outport  Port=7
  uwsCG : Outport  Port=8
  B_FM : Outport  Port=9
  wires:
  beta_wave/1 -> Wave Particle Motions/9(beta_wave)
  phi_wave/1 -> Wave Particle Motions/8(phi_wave)
  dX_CTRL/1 -> Wave Particle Motions/7(dX_CTRL)
  Cvm*dm/1 -> MATLAB Function/2(cvm)
  Wave Particle Motions/5(B_FM) -> B_FM/1
  Derivative1/1 -> MATLAB Function/3(Awrs)  "d/dt(aw-ar)"
  Add/1 -> Derivative1/1
  Wave Particle Motions/3(urs) -> Add/2
  Wave Particle Motions/2(uws) -> Add/1
  Wave Particle Motions/6(uwsCG) -> uwsCG/1
  Wave Particle Motions/4(uwXis) -> uwsXi/1
  Demux1/3 -> Nvm/1
  Demux1/1 -> Kvm/1
  Demux1/2 -> Mvm/1
  Demux/3 -> Zvm/1
  Demux/2 -> Yvm/1
  Demux/1 -> Xvm/1
  MATLAB Function/2(Mvm) -> Demux1/1  "Mvm"
  MATLAB Function/1(Fvm) -> Demux/1  "Fvm"
  Bv_ship/1 -> Wave Particle Motions/1(U_ship)
  dLCG/1 -> Wave Particle Motions/6(dLCG)
  SeaState/1 -> Wave Particle Motions/5(SeaState)
  Wave Particle Motions/1(Rs) -> MATLAB Function/1(Rs)
  CG/1 -> Wave Particle Motions/4(CG)
  CGi/1 -> Wave Particle Motions/3(CGi)
  Bx_earth/1 -> Wave Particle Motions/2(X_earth)

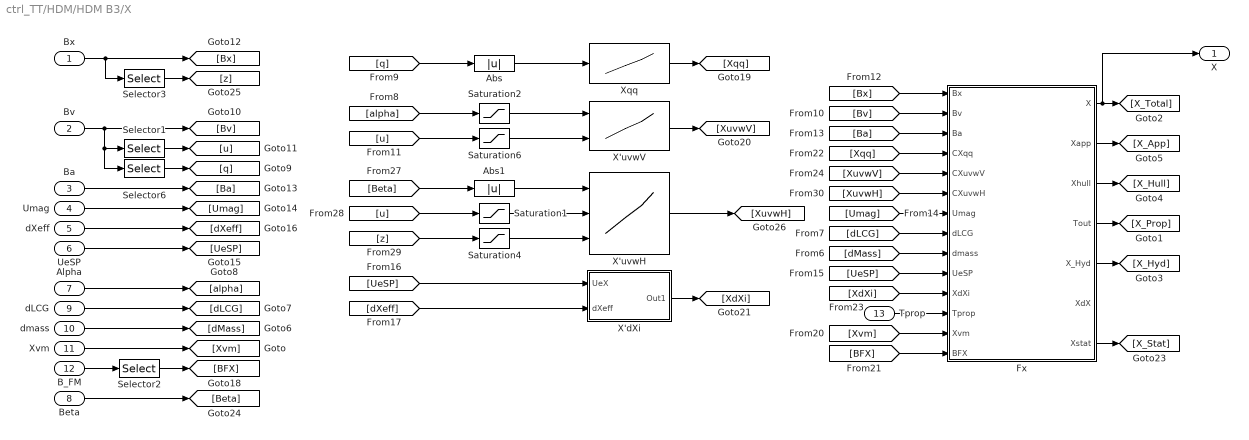
== system ctrl_TT/HDM/HDM B3/X ==
  Bx : Inport
  Bv : Inport  Port=2
  Ba : Inport  Port=3
  Umag : Inport  Port=4
  dXeff : Inport  Port=5
  UeSP : Inport  Port=6
  Alpha : Inport  Port=7
  Beta : Inport  Port=8
  dLCG : Inport  Port=9
  dmass : Inport  Port=10
  Xvm : Inport  Port=11
  B_FM : Inport  Port=12
  Tprop : Inport  Port=13
  Abs : Abs  SaturateOnIntegerOverflow=off
  Abs1 : Abs  SaturateOnIntegerOverflow=off
  Fx : MATLAB Function  TreatAsAtomicUnit=on
  Saturation1 : Saturate  UpperLimit=-1.543332  LowerLimit=-5.14444
  Saturation2 : Saturate  UpperLimit=30  LowerLimit=-30
  Saturation4 : Saturate  UpperLimit=-13.8724  LowerLimit=-35.0624
  Saturation6 : Saturate  UpperLimit=-1.543332  LowerLimit=-5.14444
  Selector1 : Selector  InputPortWidth=6  IndexOptions=Index vector (dialog)  Indices=1  OutputSizes=1
  Selector2 : Selector  InputPortWidth=6  IndexOptions=Index vector (dialog)  Indices=1  OutputSizes=1
  Selector3 : Selector  InputPortWidth=6  IndexOptions=Index vector (dialog)  Indices=3  OutputSizes=1
  Selector6 : Selector  InputPortWidth=6  IndexOptions=Index vector (dialog)  Indices=5  OutputSizes=1
  X'dXi : Subsystem
  X'uvwH : Lookup_n-D  NumberOfTableDimensions=3  BreakpointsForDimension1=|  BreakpointsForDimension2=|  BreakpointsForDimension3=|  Table=|  InternalRulePriority=Speed  RndMeth=Simplest
      BreakpointsForDimension1=|
      | [0
      | 4
      | 8
      | 12]
      BreakpointsForDimension2=|
      | [-5.1444
      | -3.08664
      | -1.54332]
      Table=|
      | reshape([0.0000000E+00
      | 8.7490400E-05
      | -4.2970032E-04
      | -8.6882993E-04
      | 0.0000000E+00
      | 9.2255510E-05
      | -3.6462757E-04
      | -8.6516720E-04
      | 0.0000000E+00
      | -8.0508235E-05
      | -3.3610820E-04
      | -9.1603355E-04
      | 0.0000000E+00
      | -9.0915847E-05
      | -3.9252667E-04
      | -9.2068441E-04
      | 0.0000000E+00
      | -1.0407599E-04
      | -3.8836462E-04
      | -9.1865822E-04
      | 0.0000000E+00
      | -8.4723950E-05
      | -3.5324770E-04
      | -9.7126434E-04
      | 0.0000000E+00
      | -9.3766627E-05
      | -4.1342843E-04
      | -9.4161914E-04
      | 0.0000000E+00
      | -1.0916277E-04
      | -4.0683220E-04
      | -9.6707684E-04
      | 0.0000000E+00
      | -8.8664811E-05
      | -3.7605406E-04
      | -9.4194453E-04
      | 0.0000000E+00
      | -9.2876985E-05
      | -4.0365964E-04
      | -9.3239814E-04
      | 0.0000000E+00
      | -1.1414747E-04
      | -4.4323139E-04
      | -1.0049645E-03
      | 0.0000000E+00
      | -9.4615234E-05
      | -4.9251136E-04
      | -9.8471513E-04],[4,3,4])
      BreakpointsForDimension3=|
      | [-35.0624 -18.3724 -15.3724 -13.8724
      | ]
      settings: InputPortMap=u0,u1,u2
  X'uvwV : Lookup_n-D  BreakpointsForDimension1=|  BreakpointsForDimension2=|  Table=|  InternalRulePriority=Speed  RndMeth=Simplest
      BreakpointsForDimension1=|
      | [-12
      | -8
      | -4
      | 0
      | 4
      | 8
      | 12]
      BreakpointsForDimension2=|
      | [-5.1444
      | -3.08664
      | -1.54332]
      Table=|
      | reshape([8.5556500E-04
      | 9.0045500E-04
      | 9.7379500E-04
      | 1.0292250E-03
      | 1.0286950E-03
      | 9.7963500E-04
      | 1.0147450E-03
      | 9.0637500E-04
      | 9.3710500E-04
      | 1.0133950E-03
      | 1.0723650E-03
      | 1.0693650E-03
      | 1.0284650E-03
      | 1.1084650E-03
      | 9.8653120E-04
      | 9.9350120E-04
      | 1.0534412E-03
      | 1.1098412E-03
      | 1.1115412E-03
      | 1.0836412E-03
      | 1.1582412E-03],[7,3])
      settings: InputPortMap=u0,u1
  Xqq : Lookup_n-D  NumberOfTableDimensions=1  BreakpointsForDimension1=|  Table=|  InternalRulePriority=Speed  RndMeth=Simplest
      BreakpointsForDimension1=|
      | [-0.02
      | -0.015
      | -0.012958963
      | -0.009719222
      | -0.006479482
      | -0.003239741
      | -0.00161987
      | -0.000647948
      | 0.000647948
      | 0.00161987
      | 0.003239741
      | 0.006479482
      | 0.009719222
      | 0.012958963
      | 0.015
      | 0.02
      | ]
      Table=|
      | [1.5581E-04
      | 1.1369E-04
      | 2.0348E-04
      | 4.5268E-04
      | 3.8456E-04
      | 9.9241E-05
      | 3.8998E-04
      | 9.1300E-05
      | -3.1574E-04
      | -7.9139E-05
      | -9.0517E-04
      | -4.4764E-04
      | -5.9612E-04
      | -5.5873E-04
      | -5.9343E-04
      | -5.5869E-04
      | ]
  X : Outport
  wires:
  [XuvwH] -> Fx/6(CXuvwH)
  X'uvwH/1 -> [XuvwH]
  Saturation4/1 -> X'uvwH/3
  [z] -> Saturation4/1
  Selector3/1 -> [z]
  Saturation1/1 -> X'uvwH/2
  [u] -> Saturation1/1
  [Beta] -> Abs1/1
  Abs1/1 -> X'uvwH/1
  Beta/1 -> [Beta]
  Tprop/1 -> Fx/12(Tprop)
  [XuvwV] -> Fx/5(CXuvwV)
  [XdXi] -> Fx/11(XdXi)
  X'dXi/1(Out1) -> [XdXi]
  X'uvwV/1 -> [XuvwV]
  Xqq/1 -> [Xqq]
  [Xqq] -> Fx/4(CXqq)
  [BFX] -> Fx/14(BFX)
  Selector2/1 -> [BFX]
  [Xvm] -> Fx/13(Xvm)
  Xvm/1 -> [Xvm]
  dXeff/1 -> [dXeff]
  [dXeff] -> X'dXi/2(dXeff)
  [UeSP] -> X'dXi/1(UeX)
  UeSP/1 -> [UeSP]
  [UeSP] -> Fx/10(UeSP)
  Umag/1 -> [Umag]
  [Umag] -> Fx/7(Umag)
  Ba/1 -> [Ba]
  [Ba] -> Fx/3(Ba)
  Bx/1 -> Selector3/1, [Bx]
  [Bx] -> Fx/1(Bx)
  Selector1/1 -> [u]
  [u] -> Saturation6/1
  [Bv] -> Fx/2(Bv)
  Selector6/1 -> [q]
  Bv/1 -> Selector1/1, Selector6/1, [Bv]
  Alpha/1 -> [alpha]
  [alpha] -> Saturation2/1
  dLCG/1 -> [dLCG]
  [dLCG] -> Fx/8(dLCG)
  dmass/1 -> [dMass]
  [dMass] -> Fx/9(dmass)
  Fx/2(Xapp) -> [X_App]
  Fx/3(Xhull) -> [X_Hull]
  Fx/5(X_Hyd) -> [X_Hyd]
  Fx/4(Tout) -> [X_Prop]
  Fx/7(Xstat) -> [X_Stat]
  B_FM/1 -> Selector2/1
  Saturation6/1 -> X'uvwV/2
  Abs/1 -> Xqq/1
  [q] -> Abs/1
  Fx/1(X) -> X/1, [X_Total]
  Saturation2/1 -> X'uvwV/1
